simulink model "elevateur_NL_BF"  (R2022b)
settings: Solver=ode45  StartTime=0.0  StopTime=10  RelTol=1e-3  EnableMultiTasking=on
undefined symbols (not defined in the file): Bt, J, Ka, Kd, Ki, Kp, tau
libraries: simulink x1
settings Model: Creator=Administrateur  LastModifiedBy=dsaussie
settings SolverCC: AlgebraicLoopSolver=TrustRegion
settings DataIOCC: LimitDataPoints=on  SaveFormat=Array  SignalLoggingSaveFormat=ModelDataLogs  ReturnWorkspaceOutputs=off
settings OptimizationCC: ExpressionDepthLimit=2147483647  InitFltsAndDblsToZero=on  LifeSpan=inf
settings DebuggingCC: UnderspecifiedInitializationDetection=Classic  MergeDetectMultiDrivingBlocksExec=none  SolverPrmCheckMsg=warning  UnconnectedInputMsg=warning  UnconnectedOutputMsg=warning  UnconnectedLineMsg=warning  AllowSymbolicDim=off  StateNameClashWarn=warning  SFUnexpectedBacktrackingDiag=warning  SFNoUnconditionalDefaultTransitionDiag=warning  SFExecutionAtInitializationDiag=none  SFMachineParentedDataDiag=warning  ArithmeticOperatorsInVariantConditions=warning
settings HardwareCC: ProdBitPerPointer=32  ProdBitPerSizeT=32  ProdBitPerPtrDiffT=32  ProdLargestAtomicFloat=None  ProdIntDivRoundTo=Undefined  ProdEndianess=Unspecified  ProdWordSize=32  ProdHWDeviceType=32-bit Generic
settings ModelReferenceCC: EnableRefExpFcnMdlSchedulingChecks=on  PropagateSignalLabelsOutOfModel=off
settings SFSimCC: SimUseLocalCustomCode=off  CustomCodeUndefinedFunction=UseInterfaceOnly
settings RTWCC: RTWUseLocalCustomCode=off
settings CodeAppCC: StateflowObjectComments=on
settings GRTTargetCC: TargetLangStandard=C89/C90 (ANSI)  CombineOutputUpdateFcns=off  GRTInterface=on
settings ConfigComp: CovMetricSettings=dw  CovSaveCumulativeToWorkspaceVar=on  CovSaveSingleToWorkspaceVar=on  CovExternalEMLEnable=off

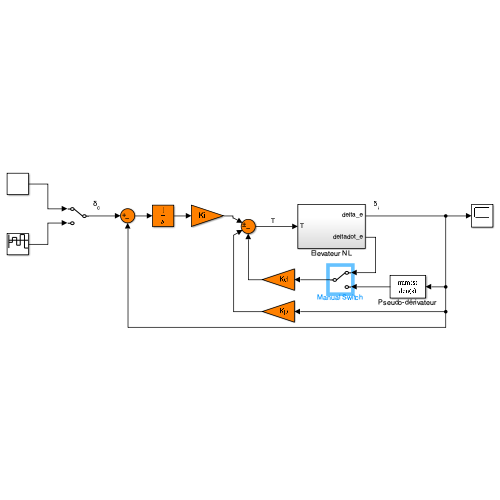
[thumbnail: Simulink's stored preview of the top-level diagram]
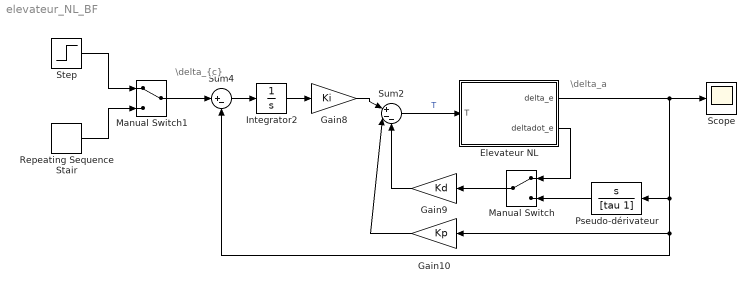
== system elevateur_NL_BF ==
  note: \delta_a
  note: \delta_{c}
  Elevateur NL : Subsystem
  Gain10 : Gain  Gain=Kp
  Gain8 : Gain  Gain=Ki
  Gain9 : Gain  Gain=Kd
  Integrator2 : Integrator
  Manual Switch : ManualSwitch
  Manual Switch1 : ManualSwitch
  Pseudo-dérivateur : TransferFcn  Numerator=[1 0]  Denominator=[tau 1]
  Repeating Sequence Stair : simulink/Sources/Repeating Sequence Stair  OutValues=[-0.1 0.1 -0.2 0.2 -0.3].'  tsamp=1  OutMin=[]  OutMax=[]  OutDataTypeStr=double  OutputDataTypeScalingMode=double  OutDataType=fixdt(0,8)  ConRadixGroup=Best Precision: Vector-wise  OutScaling=2^-12
  Scope : Scope
  Step : Step  Time=0  SampleTime=0
  Sum2 : Sum  Inputs=|+--
  Sum4 : Sum  Inputs=|+-
  wires:
  Gain10/1 -> Sum2/2
  Gain9/1 -> Sum2/3
  Gain8/1 -> Sum2/1
  Integrator2/1 -> Gain8/1
  Sum4/1 -> Integrator2/1
  Sum2/1 -> Elevateur NL/1(T)  "T"
  Elevateur NL/1(delta_e) -> Pseudo-dérivateur/1, Gain10/1, Sum4/2, Scope/1
  Pseudo-dérivateur/1 -> Manual Switch/2
  Manual Switch/1 -> Gain9/1
  Elevateur NL/2(deltadot_e) -> Manual Switch/1
  Manual Switch1/1 -> Sum4/1
  Step/1 -> Manual Switch1/1
  Repeating Sequence Stair/1 -> Manual Switch1/2

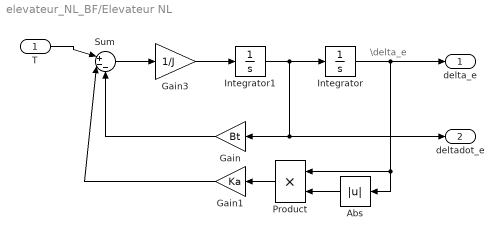
== system elevateur_NL_BF/Elevateur NL ==
  note: \delta_e
  T : Inport
  Abs : Abs  SaturateOnIntegerOverflow=off
  Gain : Gain  Gain=Bt
  Gain1 : Gain  Gain=Ka
  Gain3 : Gain  Gain=1/J
  Integrator : Integrator
  Integrator1 : Integrator
  Product : Product
  Sum : Sum  Inputs=|+--
  delta_e : Outport  VectorParamsAs1DForOutWhenUnconnected=off
  deltadot_e : Outport  Port=2  VectorParamsAs1DForOutWhenUnconnected=off
  wires:
  Gain3/1 -> Integrator1/1
  Integrator1/1 -> Integrator/1, Gain/1, deltadot_e/1
  Sum/1 -> Gain3/1
  Gain/1 -> Sum/3
  Gain1/1 -> Sum/2
  T/1 -> Sum/1
  Abs/1 -> Product/2
  Integrator/1 -> Abs/1, Product/1, delta_e/1
  Product/1 -> Gain1/1
